simulink model "doublerotor"  (R2020a)
settings: Solver=VariableStepAuto  StartTime=0.0  StopTime=10.0  RelTol=1e-3  EnableMultiTasking=on
values from neighbouring files (symbols this model uses):
  A = [ 0 1 0 0 0 0 ... (first row only)    [main.m]    (also in proje1.m)
  B = [0 0 ... (first row only)    [main.m]    (also in proje1.m)
  K = place(A,B,p)    [main.m]    (also in proje1.m)
settings Model: Creator=Nariman  LastModifiedBy=Nariman
settings DataIOCC: ReturnWorkspaceOutputs=off
settings OptimizationCC: LifeSpan=inf
settings DebuggingCC: SFUnexpectedBacktrackingDiag=warning  SFNoUnconditionalDefaultTransitionDiag=warning  ArithmeticOperatorsInVariantConditions=warning
settings SFSimCC: SimUseLocalCustomCode=off  CustomCodeUndefinedFunction=UseInterfaceOnly
settings RTWCC: RTWUseLocalCustomCode=off
settings CodeAppCC: StateflowObjectComments=on
settings GRTTargetCC: TargetLangStandard=C89/C90 (ANSI)
settings ConfigComp: CovMetricSettings=dw  CovHtmlReporting=on  CovSaveCumulativeToWorkspaceVar=on  CovSaveSingleToWorkspaceVar=on  CovExternalEMLEnable=off

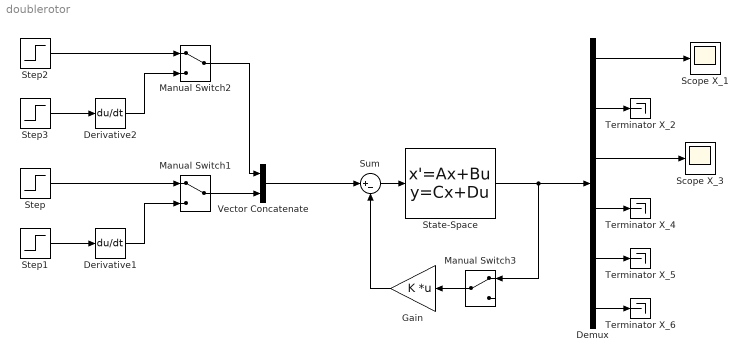
== system doublerotor ==
  Demux : Demux  Outputs=6
  Derivative1 : Derivative
  Derivative2 : Derivative
  Gain : Gain  Gain=K  Multiplication=Matrix(K*u)
  Manual Switch1 : ManualSwitch
  Manual Switch2 : ManualSwitch
  Manual Switch3 : ManualSwitch
  "Scope X_1 " : Scope
  Scope X_3 : Scope
  State-Space : StateSpace  A=A  B=B  C=eye(6)  D=zeros(6,2)  InitialCondition=0
  Step : Step  After=100  SampleTime=0
  Step1 : Step  Time=4  SampleTime=0
  Step2 : Step  After=10  SampleTime=0
  Step3 : Step  Time=4  SampleTime=0
  Sum : Sum  Inputs=|+-
  Terminator X_{2,4..6} (4 alike) : Terminator
  Vector Concatenate : Concatenate  Mode=Multidimensional array
  wires:
  Step/1 -> Manual Switch1/1
  Derivative1/1 -> Manual Switch1/2
  Step1/1 -> Derivative1/1
  Demux/1 -> "Scope X_1 "/1
  Manual Switch1/1 -> Vector Concatenate/2
  Step2/1 -> Manual Switch2/1
  Derivative2/1 -> Manual Switch2/2
  Step3/1 -> Derivative2/1
  Manual Switch2/1 -> Vector Concatenate/1
  Sum/1 -> State-Space/1
  Gain/1 -> Sum/2
  State-Space/1 -> Manual Switch3/1, Demux/1
  Vector Concatenate/1 -> Sum/1
  Demux/3 -> Scope X_3/1
  Demux/2 -> Terminator X_2/1
  Demux/4 -> Terminator X_4/1
  Demux/6 -> Terminator X_6/1
  Demux/5 -> Terminator X_5/1
  Manual Switch3/1 -> Gain/1
